simulink library "Volume"  (R2022b)
settings: Solver=VariableStepAuto  StartTime=0.0  StopTime=10.0  RelTol=1e-3
libraries: VolumeBtc x1
settings Model: Creator=kl13806  LastModifiedBy=kl13806
settings SolverCC: AlgebraicLoopSolver=TrustRegion
settings DebuggingCC: UnconnectedInputMsg=warning  UnconnectedOutputMsg=warning  UnconnectedLineMsg=warning  SFMachineParentedDataDiag=warning  ArithmeticOperatorsInVariantConditions=warning
settings ModelReferenceCC: EnableRefExpFcnMdlSchedulingChecks=on
settings SFSimCC: SimUseLocalCustomCode=off  CustomCodeUndefinedFunction=UseInterfaceOnly
settings RTWCC: RTWUseLocalCustomCode=off  DLArmComputeVersion=19.05

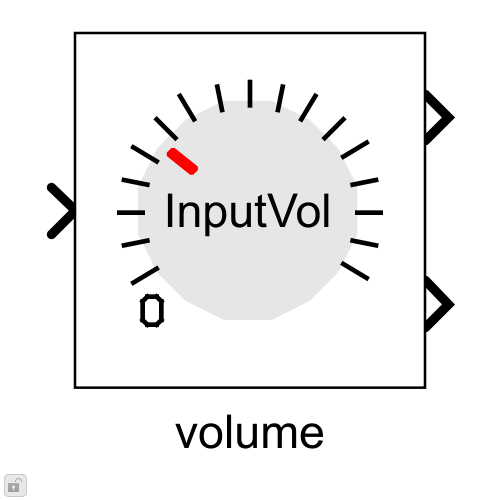
[thumbnail: Simulink's stored preview of the top-level diagram]
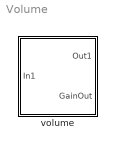
== system Volume ==
  volume : Subsystem  mask(Bose Audio Volume){FeatureName=InputVol, initial_linear_gain=0, MaskEnableGainOutput=on, MaskRows=8, MaskVolumeTable=[0 -100; 0.5 -30; 1 0], BankNumber=0, TriggerInit=[140 80 220 140]}
      mask prompts: FeatureName "Signal Name (controls FeaturePath)"; initial_linear_gain "Initial gain (linear)"; MaskEnableGainOutput "Enable output gain port"; MaskRows "Maximum Table Points"; MaskVolumeTable "Default Table"; BankNumber "Memory Bank Number:"; TriggerInit "Hidden: MoveFcn redraw"
      mask help: This volume signal block includes receipt of volume level (via RTC) as well as tuning variables to calibrate a gain table that maps 8-bit integer volume index (from RTC) to float decibels.
      mask init:
      | blkh = gcbh;
      | % Copy discrete mask parameters into a classdef object
      | InnerLinkConfig = VolumeConfig;
      | InnerLinkConfig.InitialLinearGain = initial_linear_gain;
      | InnerLinkConfig.MaskEnableGainOutput = MaskEnableGainOutput;
      | InnerLinkConfig.MaskRows = MaskRows;
      | InnerLinkConfig.MaskVolumeTable = MaskVolumeTable;
      | InnerLinkConfig.BankNumber = BankNumber;
      | 
      | % Hookup gain port
      | EnableBlockPort(blkh,'GainOut',MaskEnableGainOutput);
      settings: MoveFcn=VolumeMask.CB_TriggerInit(gcbh);
      mask Help:
      | This block allows a ramped change in volume using rgainy block.
      | - The initial gain to be applied to the input audio can be set (typically 0)
      | 
      | RTC CONTROL:
      | Run time control is available to dynamically mute the audio. The volume index can be provided (typically between 0-255), along with a ramp time and rate (rate gets precedence).
      | RTC_SIM_OBJ.AddREQ( 'VolumeSet', 0.6, [0005,  <volume_index>, <ramp_db_per_second>, <ramp_time>]);
      | E.g., RTC_SIM_OBJ.AddREQ( 'VolumeSet', 0.7, [0005, 255, 0, 50]);
      mask TypeOptions FeatureName: InnerLink/FeatureName
      mask Callback TriggerInit: VolumeMask.CB_TriggerInit(gcbh);
      mask DialogControl CalibrationGroup Prompt: Signal Calibration
      mask Display:
      | [path,w,h] = IconVolumeMask();
      | 
      | % work in pixels since the icon does not scale
      | pos = get(gcbh,'position');
      | bw = pos(3) - pos(1);
      | bh = pos(4) - pos(2);
      | 
      | % Draw centered icon
      | xAdj = bw/2 - w/2;
      | yAdj = bh/2 - h/2;
      | for i=1:length(path)
      |     if (path(i).rgb(1) >= 0)
      |         patch(path(i).x+xAdj, path(i).y+yAdj, path(i).rgb);
      |     end
      |     if (path(i).stroke(1) >= 0)
      |         plot(path(i).x+xAdj, path(i).y+yAdj);
      |     end
      | end
      | 
      | % Display some text
      | text(bw/2, bh/2,FeatureName, ...
      |     'horizontalAlignment','center', ...
      |     'VerticalAlignment','middle');

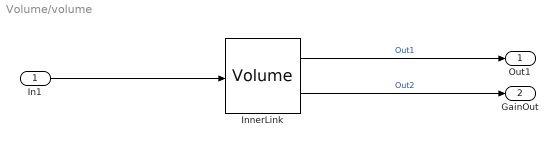
== system Volume/volume ==
  In1 : Inport
  InnerLink : VolumeBtc/Volume  FeatureName=InputVol  Config=InnerLinkConfig  EnableGainOut=on  TriggerInit=[60 35 135 110]
      settings: SourceProductName=Bose Blocklib
  Out1 : Outport
  GainOut : Outport  Port=2
  wires:
  InnerLink/1 -> Out1/1  "Out1"
  InnerLink/2 -> GainOut/1  "Out2"
  In1/1 -> InnerLink/1
